simulink model "robot_LAB__3_2"  (R2024b)
settings: Solver=VariableStepAuto  StartTime=0.0  StopTime=T_SIM  RelTol=1e-3
values from neighbouring files (symbols this model uses):
  d = 0.165    [init_LAB__3.m]
  diff_flatness = 0    [init_LAB__3.m]
  k_sign = sign(k_i)    [init_LAB__3.m]
  q_i = [-0.5, -0.5, pi/2]    [init_LAB__3.m]
  r = 0.03    [init_LAB__3.m]
  t_law = 1    [init_LAB__3.m]
  Ta = 1    [MAIN_ROBOT.m]    (also in init_LAB__2.m; init_LAB__3.m)
  Tc = 30    [MAIN_ROBOT.m]    (also in init_LAB__2.m; init_LAB__3.m = 45)
  y = R*sin(omega_trj.*s)    [MAIN_ROBOT.m]    (also in init_LAB__2.m; init_LAB__3.m = planTrajectoryChainedForm(q_i, q_f, reorientation))
settings Model: Creator=leontecosm  LastModifiedBy=Enrico

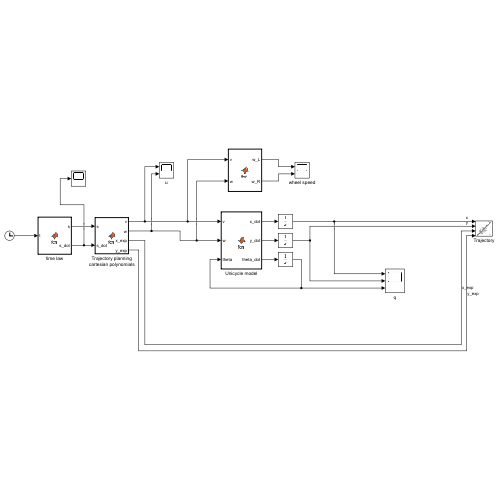
[thumbnail: Simulink's stored preview of the top-level diagram]
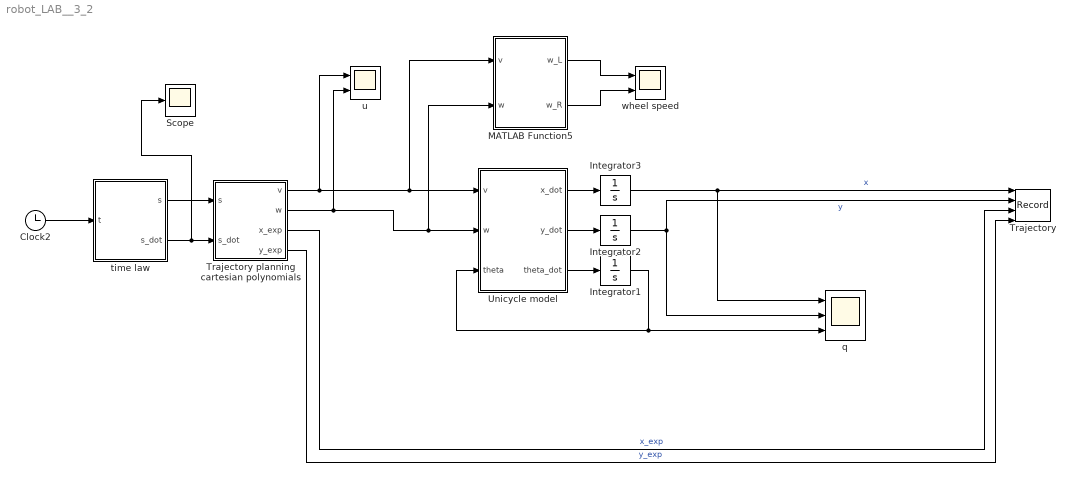
== system robot_LAB__3_2 ==
  Clock2 : Clock
  Integrator1 : Integrator  InitialCondition=q_i(3)
  Integrator2 : Integrator  InitialCondition=q_i(2)
  Integrator3 : Integrator  InitialCondition=q_i(1)
  MATLAB Function5 : MATLAB Function  TreatAsAtomicUnit=on
  Scope : Scope
  Trajectory : Record  FileSettingsInternal="{\"entries\":[{\"content\":{\"excelSettings\":{\"content\":{},\"type\":\"Streamout.ExcelSettings\"}},\"type\":\"Streamout.FileSettingStorage\",\"uuid\":\"\"}],\"packageUris\":[\"http:\\/\\/schema.mathworks.com\\/mf0\\/streamout_blocks\\/R2020a\"],\"version\":\"1.0\"}"  Layout=[1 1]  SignalsInternal="{\"entries\":[{\"content\":{\"signals\":[{\"content\":{\"blockPath\":[],\"dimensions\":[1],\"domain\":\"\",\"lineColor\":\"#a2142f\",\"plots\":[ 1 ],\"port\":1,\"sid\":[\"\"],\"signalID\":1,\"signalName\":\"x\"},\"type\":\"RecordBlkView.Signal\",\"uuid\":\"\"},{\"content\":{\"blockPath\":[],\"dimensions\":[1],\"domain\":\"\",\"lineColor\":\"#fe330a\",\"plots\":[ 1 ],\"port\":2,\"sid\":[\"\"],\"signalID\":2,\"signalName\":\"y\"},\"type\":\"RecordBlkView.Signal\",\"uuid\":\"\"},{\"content\":{\"blockPath\":[],\"dimensions\":[1],\"domain\":\"\",\"lineColor\":\"#77ac30\",\"lineWidth\":2,\"plots\":[ 1 ],\"port\":3,\"sid\":[\"\"],\"signalID\":3,\"signalName\":\"x_exp\"},\"type\":\"RecordBlkView.Signal\",\"uuid\":\"\"},{\"content\":{\"blockPath\":[],\"dimensions\":[1],\"domain\":\"\",\"lineColor\":\"#64d413\",\"lineWidth\":2,\"plots\":[ 1 ],\"port\":4,\"sid\":[\"\"],\"signalID\":4,\"signalName\":\"y_exp\"},\"type\":\"RecordBlkView.Signal\",\"uuid\":\"\"}]},\"type\":\"RecordBlkView.InputSignals\",\"uuid\":\"\"}],\"packageUris\":[\"http:\\/\\/schema.mathworks.com\\/mf0\\/streamout_blocks\\/R2020a\"],\"version\":\"1.0\"}"  VisualizationBindings="{\"xyplotplugin\":{\"info\":[{\"series\":[{\"bindingParametersList\":[{\"parameter\":\"X-Axis\",\"signalID\":1,\"signalName\":\"x\"},{\"parameter\":\"Y-Axis\",\"signalID\":2,\"signalName\":\"y\"},{\"parameter\":\"X-Axis\",\"signalID\":1,\"signalName\":\"x\"},{\"parameter\":\"Y-Axis\",\"signalID\":2,\"signalName\":\"y\"}],\"seriesID\":0},{\"bindingParametersList\":[{\"parameter\":\"X-Axis\",\"signalID\":3,\"signalName\":\"x_exp\"},{\"parameter\":\"Y-Axis\",\"signalID\":4,\"signalName\":\"y_exp\"}],\"seriesID\":1}],\"subplotID\":1}]}}"  CompatibilityTag=XY
  Trajectory planning cartesian polynomials : MATLAB Function  TreatAsAtomicUnit=on
  Unicycle model : MATLAB Function  TreatAsAtomicUnit=on
  q : Scope  NumInputPorts=3
  time law : MATLAB Function  TreatAsAtomicUnit=on
  u : Scope  NumInputPorts=2
  wheel speed : Scope  NumInputPorts=2
  wires:
  Integrator1/1 -> Unicycle model/3(theta), q/3
  Unicycle model/1(x_dot) -> Integrator3/1
  time law/1(s) -> Trajectory planning cartesian polynomials/1(s)
  Integrator3/1 -> q/1, Trajectory/1  "x"
  MATLAB Function5/1(w_L) -> wheel speed/1
  Trajectory planning cartesian polynomials/2(w) -> u/2, MATLAB Function5/2(w), Unicycle model/2(w)
  Trajectory planning cartesian polynomials/4(y_exp) -> Trajectory/4  "y_exp"
  MATLAB Function5/2(w_R) -> wheel speed/2
  Trajectory planning cartesian polynomials/3(x_exp) -> Trajectory/3  "x_exp"
  Unicycle model/2(y_dot) -> Integrator2/1
  Integrator2/1 -> Trajectory/2, q/2  "y"
  Trajectory planning cartesian polynomials/1(v) -> u/1, Unicycle model/1(v), MATLAB Function5/1(v)
  Unicycle model/3(theta_dot) -> Integrator1/1
  time law/2(s_dot) -> Scope/1, Trajectory planning cartesian polynomials/2(s_dot)
  Clock2/1 -> time law/1(t)

== matlab function robot_LAB__3_2/Trajectory planning cartesian polynomials ==
  data: s input; v output; s_dot input; w output; y parameter; k_sign parameter; x_exp output; y_exp output; diff_flatness parameter
function [v,w,x_exp,y_exp] = fcn(s, s_dot, y, k_sign, diff_flatness)

    if (diff_flatness == 0)

        x_exp = y(1,1) * s^3 - y(1,2) * (s - 1)^3 + y(1,3) * s^2 * (s - 1) + y(1,4) * s * (s - 1)^2;
        y_exp = y(2,1) * s^3 - y(2,2) * (s - 1)^3 + y(2,3) * s^2 * (s - 1) + y(2,4) * s * (s - 1)^2;

        x_dot = 3 * y(1,1) * s^2 - 3 * y(1,2) * (s-1)^2 + 2 * y(1,3) * s * (s-1) + y(1,3) * s^2 + y(1,4) * (s-1)^2 + 2 * y(1,4) * s * (s-1);
        y_dot = 3 * y(2,1) * s^2 - 3 * y(2,2) * (s-1)^2 + 2 * y(2,3) * s * (s-1) + y(2,3) * s^2 + y(2,4) * (s-1)^2 + 2 * y(2,4) * s * (s-1);
        x_dotdot = 6 * y(1,1) * s - 6 * y(1,2) * (s-1) + 2 * y(1,3) * s + 2 * y(1,3) * (s-1) + 2 * s * y(1,3) + 2 * y(1,4) * (s-1) + 2 * y(1,4) * s + 2 * y(1,4) * (s-1);
        y_dotdot = 6 * y(2,1) * s - 6 * y(2,2) * (s-1) + 2 * y(2,3) * s + 2 * y(2,3) * (s-1) + 2 * s * y(2,3) + 2 * y(2,4) * (s-1) + 2 * y(2,4) * s + 2 * y(2,4) * (s-1);
    
    
        if(k_sign == 1)
            v = sqrt((x_dot)^2 + (y_dot)^2) * s_dot;
        else
            v = - sqrt((x_dot)^2 + (y_dot)^2) * s_dot;
        end

        w = (((x_dot) * (y_dotdot) - (y_dot) * (x_dotdot)) / ((x_dot)^2 + (y_dot)^2)) * s_dot;
     
    else 

            z1 = y(1,1) * s - y(1,2) * (s - 1);
            z3 = y(2,1) * s^3 - y(2,2) * (s - 1)^3 + y(2,3) * s^2 * (s - 1) + y(2,4) * s * (s - 1)^2;
            z1_dot = y(1,1) - y(1,2);
            z3_dot = 3 * y(2,1) * s^2 - 3 * y(2,2) * (s-1)^2 + 2 * y(2,3) * s * (s - 1) + y(2,3) * s^2 + y(2,4) * (s - 1)^2 + 2 * y(2,4) * s * (s - 1);
            z1_dotdot = 0;
            z3_dotdot = 6 * y(2,1) * s - 6 * y(2,2) * (s-1) + 2 * y(2,3) * s + 2 * y(2,3) * (s-1) + 2 * s * y(2,3) + 2 * y(2,4) * (s-1) + 2 * y(2,4) * s + 2 * y(2,4) * (s-1);

            z2 = z3_dot / z1_dot;
            
            y_exp = (z2 * sin(z1) / cos(z1) - z3) / (cos(z1) + sin(z1)^2 / cos(z1));
            x_exp = (z3 + y_exp * cos(z1)) / sin(z1);
    
            v1 = z1_dot;
            v2 = (-z1_dotdot * z3_dot + z1_dot * z3_dotdot) / (z1_dot)^2;

            v = (v2 + z3 * v1) * s_dot; 
            w =  v1 * s_dot;

    end
    
end

== matlab function robot_LAB__3_2/MATLAB Function5 ==
  data: v input; w_L output; w input; w_R output; r parameter; d parameter
function [w_L,w_R]= fcn(v,w,r, d)

w_L = v/r - d*w/(2*r);
w_R = v/r + d*w/(2*r);

== matlab function robot_LAB__3_2/Unicycle model ==
  data: v input; x_dot output; w input; theta input; y_dot output; theta_dot output
function  [x_dot, y_dot, theta_dot] = fcn(v,w,theta)
    
    x_dot = cos(theta) * v;
    y_dot = sin(theta) * v;
    theta_dot = w;

end

== matlab function robot_LAB__3_2/time law ==
  data: s output; t input; Ta parameter; s_dot output; Tc parameter; t_law parameter
function [s,s_dot]=fcn(t, Ta, Tc, t_law)

    v_c = 1 / (Ta + Tc);
    a = v_c / Ta;

    if (t_law == 0)
        s_dot = 1/Tc;
        s = s_dot * t;

        if(t > Tc)
            s_dot = 0;
            s = 1;
        end
    else
        if(t > 2*Ta+Tc)
            s_dot = 0;
            s = 1;
        elseif(t > Ta+Tc)
            s_dot = v_c - a * (t - Ta - Tc);
            s = (a * Ta^2)/2 + v_c * (Tc) + (a * (t - Tc - Ta)^2)/2;
        elseif(t > Ta)
            s_dot = v_c; 
            s = (a * Ta^2)/2 + v_c * (t - Ta);
        else 
            s_dot = a * t;
            s = (a * t^2)/2;
        end
    end
end
